simulink model "lo_values_test_v11"  (R2012b)
settings: Solver=ode45  StartTime=0.0  StopTime=100000  RelTol=1e-3
values from neighbouring files (symbols this model uses):
  Fs = 640e6    (= 640000000)    [filter_coefficients.m]    (also in filter_design.m; filter_design_getting_order.m)
undefined symbols (not defined in the file or in its folder): get, sided, Two
undefined symbols (not defined in the file): A_cos, A_sin, B_cos, B_sin, C_cos, C_sin, casper_coef, coef, D_cos, D_sin
libraries: xbsIndex_r4 x1768, dspsnks4 x10, casper_library_misc x9, xps_library x2, simulink x1
(part 2 of 17)

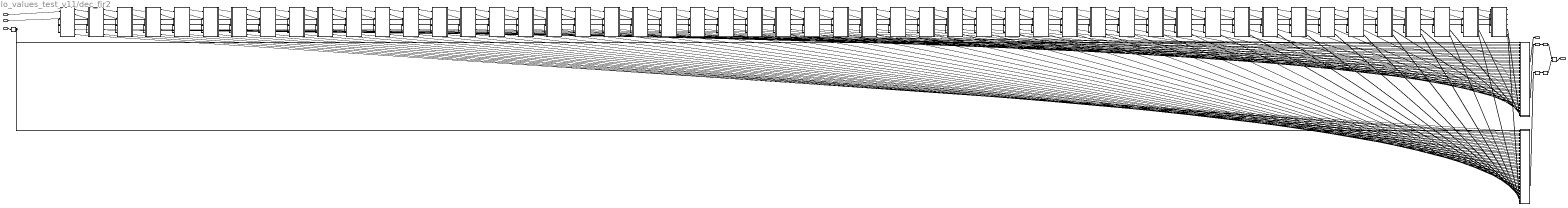
== system lo_values_test_v11/dec_fir2 ==
  sync_in : Inport
  real1 : Inport  Port=2
  imag1 : Inport  Port=3
  convert1 : xbsIndex_r4/Convert  gui_display_data_type=Fixed-point  arith_type="Signed  (2's comp)"  n_bits=16  bin_pt=15  float_type=Single  exp_bits=8  fraction_bits=24  quantization="Round  (unbiased: +/- Inf)"  overflow=Wrap  en=off  latency=2  dbl_ovrd=off  pipeline=off  block_type=convert
  convert2 : xbsIndex_r4/Convert  gui_display_data_type=Fixed-point  arith_type="Signed  (2's comp)"  n_bits=16  bin_pt=15  float_type=Single  exp_bits=8  fraction_bits=24  quantization="Round  (unbiased: +/- Inf)"  overflow=Wrap  en=off  latency=2  dbl_ovrd=off  pipeline=off  block_type=convert
  delay : xbsIndex_r4/Delay  rst=off  infoeditControl=Selection of Reset will increase slice count due to use of real FFs and instead of SRLs  en=off  latency=5  dbl_ovrd=off  reg_retiming=off  block_type=delay
  fir_dbl_col1 : Subsystem  AncestorBlock=casper_library_downconverter/fir_dbl_col  mask(fir_dbl_col){n_inputs=1, coeff=[0.00034504], add_latency=1, mult_latency=2, coeff_bit_width=25, coeff_bin_pt=24, first_stage_hdl=on, adder_imp=DSP48}
      mask prompts: n_inputs "Inputs"; coeff "Coefficients"; add_latency "Add latency"; mult_latency "Mult Latency"; coeff_bit_width "Coefficient bit width"; coeff_bin_pt "Coefficient binary point"; first_stage_hdl "Implement first stage of adder trees on output as behavioural HDL"; adder_imp "Adder implementation"
      mask init: same as lo_values_test_v11/dec_fir/fir_dbl_col1
      mask Help: eval('xlWeb(''http://casper.berkeley.edu/wiki/Fir_dbl_col'')')
      mask TypeOptions adder_imp: Behavioral | Fabric | DSP48
  fir_dbl_col10 : Subsystem  AncestorBlock=casper_library_downconverter/fir_dbl_col  mask(fir_dbl_col){n_inputs=1, coeff=[0.0011044], add_latency=1, mult_latency=2, coeff_bit_width=25, coeff_bin_pt=24, first_stage_hdl=on, adder_imp=DSP48}
      mask prompts: n_inputs "Inputs"; coeff "Coefficients"; add_latency "Add latency"; mult_latency "Mult Latency"; coeff_bit_width "Coefficient bit width"; coeff_bin_pt "Coefficient binary point"; first_stage_hdl "Implement first stage of adder trees on output as behavioural HDL"; adder_imp "Adder implementation"
      mask init: same as lo_values_test_v11/dec_fir/fir_dbl_col1
      mask Help: eval('xlWeb(''http://casper.berkeley.edu/wiki/Fir_dbl_col'')')
      mask TypeOptions adder_imp: Behavioral | Fabric | DSP48
  fir_dbl_col11 : Subsystem  AncestorBlock=casper_library_downconverter/fir_dbl_col  mask(fir_dbl_col){n_inputs=1, coeff=[0.0012861], add_latency=1, mult_latency=2, coeff_bit_width=25, coeff_bin_pt=24, first_stage_hdl=on, adder_imp=DSP48}
      mask prompts: n_inputs "Inputs"; coeff "Coefficients"; add_latency "Add latency"; mult_latency "Mult Latency"; coeff_bit_width "Coefficient bit width"; coeff_bin_pt "Coefficient binary point"; first_stage_hdl "Implement first stage of adder trees on output as behavioural HDL"; adder_imp "Adder implementation"
      mask init: same as lo_values_test_v11/dec_fir/fir_dbl_col1
      mask Help: eval('xlWeb(''http://casper.berkeley.edu/wiki/Fir_dbl_col'')')
      mask TypeOptions adder_imp: Behavioral | Fabric | DSP48
  fir_dbl_col12 : Subsystem  AncestorBlock=casper_library_downconverter/fir_dbl_col  mask(fir_dbl_col){n_inputs=1, coeff=[0.0014864], add_latency=1, mult_latency=2, coeff_bit_width=25, coeff_bin_pt=24, first_stage_hdl=on, adder_imp=DSP48}
      mask prompts: n_inputs "Inputs"; coeff "Coefficients"; add_latency "Add latency"; mult_latency "Mult Latency"; coeff_bit_width "Coefficient bit width"; coeff_bin_pt "Coefficient binary point"; first_stage_hdl "Implement first stage of adder trees on output as behavioural HDL"; adder_imp "Adder implementation"
      mask init: same as lo_values_test_v11/dec_fir/fir_dbl_col1
      mask Help: eval('xlWeb(''http://casper.berkeley.edu/wiki/Fir_dbl_col'')')
      mask TypeOptions adder_imp: Behavioral | Fabric | DSP48
  fir_dbl_col13 : Subsystem  AncestorBlock=casper_library_downconverter/fir_dbl_col  mask(fir_dbl_col){n_inputs=1, coeff=[0.0017056], add_latency=1, mult_latency=2, coeff_bit_width=25, coeff_bin_pt=24, first_stage_hdl=on, adder_imp=DSP48}
      mask prompts: n_inputs "Inputs"; coeff "Coefficients"; add_latency "Add latency"; mult_latency "Mult Latency"; coeff_bit_width "Coefficient bit width"; coeff_bin_pt "Coefficient binary point"; first_stage_hdl "Implement first stage of adder trees on output as behavioural HDL"; adder_imp "Adder implementation"
      mask init: same as lo_values_test_v11/dec_fir/fir_dbl_col1
      mask Help: eval('xlWeb(''http://casper.berkeley.edu/wiki/Fir_dbl_col'')')
      mask TypeOptions adder_imp: Behavioral | Fabric | DSP48
  fir_dbl_col14 : Subsystem  AncestorBlock=casper_library_downconverter/fir_dbl_col  mask(fir_dbl_col){n_inputs=1, coeff=[0.0019439], add_latency=1, mult_latency=2, coeff_bit_width=25, coeff_bin_pt=24, first_stage_hdl=on, adder_imp=DSP48}
      mask prompts: n_inputs "Inputs"; coeff "Coefficients"; add_latency "Add latency"; mult_latency "Mult Latency"; coeff_bit_width "Coefficient bit width"; coeff_bin_pt "Coefficient binary point"; first_stage_hdl "Implement first stage of adder trees on output as behavioural HDL"; adder_imp "Adder implementation"
      mask init: same as lo_values_test_v11/dec_fir/fir_dbl_col1
      mask Help: eval('xlWeb(''http://casper.berkeley.edu/wiki/Fir_dbl_col'')')
      mask TypeOptions adder_imp: Behavioral | Fabric | DSP48
  fir_dbl_col15 : Subsystem  AncestorBlock=casper_library_downconverter/fir_dbl_col  mask(fir_dbl_col){n_inputs=1, coeff=[0.0022021], add_latency=1, mult_latency=2, coeff_bit_width=25, coeff_bin_pt=24, first_stage_hdl=on, adder_imp=DSP48}
      mask prompts: n_inputs "Inputs"; coeff "Coefficients"; add_latency "Add latency"; mult_latency "Mult Latency"; coeff_bit_width "Coefficient bit width"; coeff_bin_pt "Coefficient binary point"; first_stage_hdl "Implement first stage of adder trees on output as behavioural HDL"; adder_imp "Adder implementation"
      mask init: same as lo_values_test_v11/dec_fir/fir_dbl_col1
      mask Help: eval('xlWeb(''http://casper.berkeley.edu/wiki/Fir_dbl_col'')')
      mask TypeOptions adder_imp: Behavioral | Fabric | DSP48
  fir_dbl_col16 : Subsystem  AncestorBlock=casper_library_downconverter/fir_dbl_col  mask(fir_dbl_col){n_inputs=1, coeff=[0.0024799], add_latency=1, mult_latency=2, coeff_bit_width=25, coeff_bin_pt=24, first_stage_hdl=on, adder_imp=DSP48}
      mask prompts: n_inputs "Inputs"; coeff "Coefficients"; add_latency "Add latency"; mult_latency "Mult Latency"; coeff_bit_width "Coefficient bit width"; coeff_bin_pt "Coefficient binary point"; first_stage_hdl "Implement first stage of adder trees on output as behavioural HDL"; adder_imp "Adder implementation"
      mask init: same as lo_values_test_v11/dec_fir/fir_dbl_col1
      mask Help: eval('xlWeb(''http://casper.berkeley.edu/wiki/Fir_dbl_col'')')
      mask TypeOptions adder_imp: Behavioral | Fabric | DSP48
  fir_dbl_col17 : Subsystem  AncestorBlock=casper_library_downconverter/fir_dbl_col  mask(fir_dbl_col){n_inputs=1, coeff=[0.0027778], add_latency=1, mult_latency=2, coeff_bit_width=25, coeff_bin_pt=24, first_stage_hdl=on, adder_imp=DSP48}
      mask prompts: n_inputs "Inputs"; coeff "Coefficients"; add_latency "Add latency"; mult_latency "Mult Latency"; coeff_bit_width "Coefficient bit width"; coeff_bin_pt "Coefficient binary point"; first_stage_hdl "Implement first stage of adder trees on output as behavioural HDL"; adder_imp "Adder implementation"
      mask init: same as lo_values_test_v11/dec_fir/fir_dbl_col1
      mask Help: eval('xlWeb(''http://casper.berkeley.edu/wiki/Fir_dbl_col'')')
      mask TypeOptions adder_imp: Behavioral | Fabric | DSP48
  fir_dbl_col18 : Subsystem  AncestorBlock=casper_library_downconverter/fir_dbl_col  mask(fir_dbl_col){n_inputs=1, coeff=[0.0030952], add_latency=1, mult_latency=2, coeff_bit_width=25, coeff_bin_pt=24, first_stage_hdl=on, adder_imp=DSP48}
      mask prompts: n_inputs "Inputs"; coeff "Coefficients"; add_latency "Add latency"; mult_latency "Mult Latency"; coeff_bit_width "Coefficient bit width"; coeff_bin_pt "Coefficient binary point"; first_stage_hdl "Implement first stage of adder trees on output as behavioural HDL"; adder_imp "Adder implementation"
      mask init: same as lo_values_test_v11/dec_fir/fir_dbl_col1
      mask Help: eval('xlWeb(''http://casper.berkeley.edu/wiki/Fir_dbl_col'')')
      mask TypeOptions adder_imp: Behavioral | Fabric | DSP48
  fir_dbl_col19 : Subsystem  AncestorBlock=casper_library_downconverter/fir_dbl_col  mask(fir_dbl_col){n_inputs=1, coeff=[0.0034322], add_latency=1, mult_latency=2, coeff_bit_width=25, coeff_bin_pt=24, first_stage_hdl=on, adder_imp=DSP48}
      mask prompts: n_inputs "Inputs"; coeff "Coefficients"; add_latency "Add latency"; mult_latency "Mult Latency"; coeff_bit_width "Coefficient bit width"; coeff_bin_pt "Coefficient binary point"; first_stage_hdl "Implement first stage of adder trees on output as behavioural HDL"; adder_imp "Adder implementation"
      mask init: same as lo_values_test_v11/dec_fir/fir_dbl_col1
      mask Help: eval('xlWeb(''http://casper.berkeley.edu/wiki/Fir_dbl_col'')')
      mask TypeOptions adder_imp: Behavioral | Fabric | DSP48
  fir_dbl_col2 : Subsystem  AncestorBlock=casper_library_downconverter/fir_dbl_col  mask(fir_dbl_col){n_inputs=1, coeff=[0.00021473], add_latency=1, mult_latency=2, coeff_bit_width=25, coeff_bin_pt=24, first_stage_hdl=on, adder_imp=DSP48}
      mask prompts: n_inputs "Inputs"; coeff "Coefficients"; add_latency "Add latency"; mult_latency "Mult Latency"; coeff_bit_width "Coefficient bit width"; coeff_bin_pt "Coefficient binary point"; first_stage_hdl "Implement first stage of adder trees on output as behavioural HDL"; adder_imp "Adder implementation"
      mask init: same as lo_values_test_v11/dec_fir/fir_dbl_col1
      mask Help: eval('xlWeb(''http://casper.berkeley.edu/wiki/Fir_dbl_col'')')
      mask TypeOptions adder_imp: Behavioral | Fabric | DSP48
  fir_dbl_col20 : Subsystem  AncestorBlock=casper_library_downconverter/fir_dbl_col  mask(fir_dbl_col){n_inputs=1, coeff=[0.003788], add_latency=1, mult_latency=2, coeff_bit_width=25, coeff_bin_pt=24, first_stage_hdl=on, adder_imp=DSP48}
      mask prompts: n_inputs "Inputs"; coeff "Coefficients"; add_latency "Add latency"; mult_latency "Mult Latency"; coeff_bit_width "Coefficient bit width"; coeff_bin_pt "Coefficient binary point"; first_stage_hdl "Implement first stage of adder trees on output as behavioural HDL"; adder_imp "Adder implementation"
      mask init: same as lo_values_test_v11/dec_fir/fir_dbl_col1
      mask Help: eval('xlWeb(''http://casper.berkeley.edu/wiki/Fir_dbl_col'')')
      mask TypeOptions adder_imp: Behavioral | Fabric | DSP48
  fir_dbl_col21 : Subsystem  AncestorBlock=casper_library_downconverter/fir_dbl_col  mask(fir_dbl_col){n_inputs=1, coeff=[0.0041621], add_latency=1, mult_latency=2, coeff_bit_width=25, coeff_bin_pt=24, first_stage_hdl=on, adder_imp=DSP48}
      mask prompts: n_inputs "Inputs"; coeff "Coefficients"; add_latency "Add latency"; mult_latency "Mult Latency"; coeff_bit_width "Coefficient bit width"; coeff_bin_pt "Coefficient binary point"; first_stage_hdl "Implement first stage of adder trees on output as behavioural HDL"; adder_imp "Adder implementation"
      mask init: same as lo_values_test_v11/dec_fir/fir_dbl_col1
      mask Help: eval('xlWeb(''http://casper.berkeley.edu/wiki/Fir_dbl_col'')')
      mask TypeOptions adder_imp: Behavioral | Fabric | DSP48
  fir_dbl_col22 : Subsystem  AncestorBlock=casper_library_downconverter/fir_dbl_col  mask(fir_dbl_col){n_inputs=1, coeff=[0.0045537], add_latency=1, mult_latency=2, coeff_bit_width=25, coeff_bin_pt=24, first_stage_hdl=on, adder_imp=DSP48}
      mask prompts: n_inputs "Inputs"; coeff "Coefficients"; add_latency "Add latency"; mult_latency "Mult Latency"; coeff_bit_width "Coefficient bit width"; coeff_bin_pt "Coefficient binary point"; first_stage_hdl "Implement first stage of adder trees on output as behavioural HDL"; adder_imp "Adder implementation"
      mask init: same as lo_values_test_v11/dec_fir/fir_dbl_col1
      mask Help: eval('xlWeb(''http://casper.berkeley.edu/wiki/Fir_dbl_col'')')
      mask TypeOptions adder_imp: Behavioral | Fabric | DSP48
  fir_dbl_col23 : Subsystem  AncestorBlock=casper_library_downconverter/fir_dbl_col  mask(fir_dbl_col){n_inputs=1, coeff=[0.0049616], add_latency=1, mult_latency=2, coeff_bit_width=25, coeff_bin_pt=24, first_stage_hdl=on, adder_imp=DSP48}
      mask prompts: n_inputs "Inputs"; coeff "Coefficients"; add_latency "Add latency"; mult_latency "Mult Latency"; coeff_bit_width "Coefficient bit width"; coeff_bin_pt "Coefficient binary point"; first_stage_hdl "Implement first stage of adder trees on output as behavioural HDL"; adder_imp "Adder implementation"
      mask init: same as lo_values_test_v11/dec_fir/fir_dbl_col1
      mask Help: eval('xlWeb(''http://casper.berkeley.edu/wiki/Fir_dbl_col'')')
      mask TypeOptions adder_imp: Behavioral | Fabric | DSP48
  fir_dbl_col24 : Subsystem  AncestorBlock=casper_library_downconverter/fir_dbl_col  mask(fir_dbl_col){n_inputs=1, coeff=[0.0053848], add_latency=1, mult_latency=2, coeff_bit_width=25, coeff_bin_pt=24, first_stage_hdl=on, adder_imp=DSP48}
      mask prompts: n_inputs "Inputs"; coeff "Coefficients"; add_latency "Add latency"; mult_latency "Mult Latency"; coeff_bit_width "Coefficient bit width"; coeff_bin_pt "Coefficient binary point"; first_stage_hdl "Implement first stage of adder trees on output as behavioural HDL"; adder_imp "Adder implementation"
      mask init: same as lo_values_test_v11/dec_fir/fir_dbl_col1
      mask Help: eval('xlWeb(''http://casper.berkeley.edu/wiki/Fir_dbl_col'')')
      mask TypeOptions adder_imp: Behavioral | Fabric | DSP48
  fir_dbl_col25 : Subsystem  AncestorBlock=casper_library_downconverter/fir_dbl_col  mask(fir_dbl_col){n_inputs=1, coeff=[0.0058219], add_latency=1, mult_latency=2, coeff_bit_width=25, coeff_bin_pt=24, first_stage_hdl=on, adder_imp=DSP48}
      mask prompts: n_inputs "Inputs"; coeff "Coefficients"; add_latency "Add latency"; mult_latency "Mult Latency"; coeff_bit_width "Coefficient bit width"; coeff_bin_pt "Coefficient binary point"; first_stage_hdl "Implement first stage of adder trees on output as behavioural HDL"; adder_imp "Adder implementation"
      mask init: same as lo_values_test_v11/dec_fir/fir_dbl_col1
      mask Help: eval('xlWeb(''http://casper.berkeley.edu/wiki/Fir_dbl_col'')')
      mask TypeOptions adder_imp: Behavioral | Fabric | DSP48
  fir_dbl_col26 : Subsystem  AncestorBlock=casper_library_downconverter/fir_dbl_col  mask(fir_dbl_col){n_inputs=1, coeff=[0.0062713], add_latency=1, mult_latency=2, coeff_bit_width=25, coeff_bin_pt=24, first_stage_hdl=on, adder_imp=DSP48}
      mask prompts: n_inputs "Inputs"; coeff "Coefficients"; add_latency "Add latency"; mult_latency "Mult Latency"; coeff_bit_width "Coefficient bit width"; coeff_bin_pt "Coefficient binary point"; first_stage_hdl "Implement first stage of adder trees on output as behavioural HDL"; adder_imp "Adder implementation"
      mask init: same as lo_values_test_v11/dec_fir/fir_dbl_col1
      mask Help: eval('xlWeb(''http://casper.berkeley.edu/wiki/Fir_dbl_col'')')
      mask TypeOptions adder_imp: Behavioral | Fabric | DSP48
  fir_dbl_col27 : Subsystem  AncestorBlock=casper_library_downconverter/fir_dbl_col  mask(fir_dbl_col){n_inputs=1, coeff=[0.0067313], add_latency=1, mult_latency=2, coeff_bit_width=25, coeff_bin_pt=24, first_stage_hdl=on, adder_imp=DSP48}
      mask prompts: n_inputs "Inputs"; coeff "Coefficients"; add_latency "Add latency"; mult_latency "Mult Latency"; coeff_bit_width "Coefficient bit width"; coeff_bin_pt "Coefficient binary point"; first_stage_hdl "Implement first stage of adder trees on output as behavioural HDL"; adder_imp "Adder implementation"
      mask init: same as lo_values_test_v11/dec_fir/fir_dbl_col1
      mask Help: eval('xlWeb(''http://casper.berkeley.edu/wiki/Fir_dbl_col'')')
      mask TypeOptions adder_imp: Behavioral | Fabric | DSP48
  fir_dbl_col28 : Subsystem  AncestorBlock=casper_library_downconverter/fir_dbl_col  mask(fir_dbl_col){n_inputs=1, coeff=[0.0072001], add_latency=1, mult_latency=2, coeff_bit_width=25, coeff_bin_pt=24, first_stage_hdl=on, adder_imp=DSP48}
      mask prompts: n_inputs "Inputs"; coeff "Coefficients"; add_latency "Add latency"; mult_latency "Mult Latency"; coeff_bit_width "Coefficient bit width"; coeff_bin_pt "Coefficient binary point"; first_stage_hdl "Implement first stage of adder trees on output as behavioural HDL"; adder_imp "Adder implementation"
      mask init: same as lo_values_test_v11/dec_fir/fir_dbl_col1
      mask Help: eval('xlWeb(''http://casper.berkeley.edu/wiki/Fir_dbl_col'')')
      mask TypeOptions adder_imp: Behavioral | Fabric | DSP48
  fir_dbl_col29 : Subsystem  AncestorBlock=casper_library_downconverter/fir_dbl_col  mask(fir_dbl_col){n_inputs=1, coeff=[0.0076755], add_latency=1, mult_latency=2, coeff_bit_width=25, coeff_bin_pt=24, first_stage_hdl=on, adder_imp=DSP48}
      mask prompts: n_inputs "Inputs"; coeff "Coefficients"; add_latency "Add latency"; mult_latency "Mult Latency"; coeff_bit_width "Coefficient bit width"; coeff_bin_pt "Coefficient binary point"; first_stage_hdl "Implement first stage of adder trees on output as behavioural HDL"; adder_imp "Adder implementation"
      mask init: same as lo_values_test_v11/dec_fir/fir_dbl_col1
      mask Help: eval('xlWeb(''http://casper.berkeley.edu/wiki/Fir_dbl_col'')')
      mask TypeOptions adder_imp: Behavioral | Fabric | DSP48
  fir_dbl_col3 : Subsystem  AncestorBlock=casper_library_downconverter/fir_dbl_col  mask(fir_dbl_col){n_inputs=1, coeff=[0.00027945], add_latency=1, mult_latency=2, coeff_bit_width=25, coeff_bin_pt=24, first_stage_hdl=on, adder_imp=DSP48}
      mask prompts: n_inputs "Inputs"; coeff "Coefficients"; add_latency "Add latency"; mult_latency "Mult Latency"; coeff_bit_width "Coefficient bit width"; coeff_bin_pt "Coefficient binary point"; first_stage_hdl "Implement first stage of adder trees on output as behavioural HDL"; adder_imp "Adder implementation"
      mask init: same as lo_values_test_v11/dec_fir/fir_dbl_col1
      mask Help: eval('xlWeb(''http://casper.berkeley.edu/wiki/Fir_dbl_col'')')
      mask TypeOptions adder_imp: Behavioral | Fabric | DSP48
  fir_dbl_col30 : Subsystem  AncestorBlock=casper_library_downconverter/fir_dbl_col  mask(fir_dbl_col){n_inputs=1, coeff=[0.0081554], add_latency=1, mult_latency=2, coeff_bit_width=25, coeff_bin_pt=24, first_stage_hdl=on, adder_imp=DSP48}
      mask prompts: n_inputs "Inputs"; coeff "Coefficients"; add_latency "Add latency"; mult_latency "Mult Latency"; coeff_bit_width "Coefficient bit width"; coeff_bin_pt "Coefficient binary point"; first_stage_hdl "Implement first stage of adder trees on output as behavioural HDL"; adder_imp "Adder implementation"
      mask init: same as lo_values_test_v11/dec_fir/fir_dbl_col1
      mask Help: eval('xlWeb(''http://casper.berkeley.edu/wiki/Fir_dbl_col'')')
      mask TypeOptions adder_imp: Behavioral | Fabric | DSP48
  fir_dbl_col31 : Subsystem  AncestorBlock=casper_library_downconverter/fir_dbl_col  mask(fir_dbl_col){n_inputs=1, coeff=[0.0086376], add_latency=1, mult_latency=2, coeff_bit_width=25, coeff_bin_pt=24, first_stage_hdl=on, adder_imp=DSP48}
      mask prompts: n_inputs "Inputs"; coeff "Coefficients"; add_latency "Add latency"; mult_latency "Mult Latency"; coeff_bit_width "Coefficient bit width"; coeff_bin_pt "Coefficient binary point"; first_stage_hdl "Implement first stage of adder trees on output as behavioural HDL"; adder_imp "Adder implementation"
      mask init: same as lo_values_test_v11/dec_fir/fir_dbl_col1
      mask Help: eval('xlWeb(''http://casper.berkeley.edu/wiki/Fir_dbl_col'')')
      mask TypeOptions adder_imp: Behavioral | Fabric | DSP48
  fir_dbl_col32 : Subsystem  AncestorBlock=casper_library_downconverter/fir_dbl_col  mask(fir_dbl_col){n_inputs=1, coeff=[0.0091195], add_latency=1, mult_latency=2, coeff_bit_width=25, coeff_bin_pt=24, first_stage_hdl=on, adder_imp=DSP48}
      mask prompts: n_inputs "Inputs"; coeff "Coefficients"; add_latency "Add latency"; mult_latency "Mult Latency"; coeff_bit_width "Coefficient bit width"; coeff_bin_pt "Coefficient binary point"; first_stage_hdl "Implement first stage of adder trees on output as behavioural HDL"; adder_imp "Adder implementation"
      mask init: same as lo_values_test_v11/dec_fir/fir_dbl_col1
      mask Help: eval('xlWeb(''http://casper.berkeley.edu/wiki/Fir_dbl_col'')')
      mask TypeOptions adder_imp: Behavioral | Fabric | DSP48
  fir_dbl_col33 : Subsystem  AncestorBlock=casper_library_downconverter/fir_dbl_col  mask(fir_dbl_col){n_inputs=1, coeff=[0.009599], add_latency=1, mult_latency=2, coeff_bit_width=25, coeff_bin_pt=24, first_stage_hdl=on, adder_imp=DSP48}
      mask prompts: n_inputs "Inputs"; coeff "Coefficients"; add_latency "Add latency"; mult_latency "Mult Latency"; coeff_bit_width "Coefficient bit width"; coeff_bin_pt "Coefficient binary point"; first_stage_hdl "Implement first stage of adder trees on output as behavioural HDL"; adder_imp "Adder implementation"
      mask init: same as lo_values_test_v11/dec_fir/fir_dbl_col1
      mask Help: eval('xlWeb(''http://casper.berkeley.edu/wiki/Fir_dbl_col'')')
      mask TypeOptions adder_imp: Behavioral | Fabric | DSP48
  fir_dbl_col34 : Subsystem  AncestorBlock=casper_library_downconverter/fir_dbl_col  mask(fir_dbl_col){n_inputs=1, coeff=[0.010073], add_latency=1, mult_latency=2, coeff_bit_width=25, coeff_bin_pt=24, first_stage_hdl=on, adder_imp=DSP48}
      mask prompts: n_inputs "Inputs"; coeff "Coefficients"; add_latency "Add latency"; mult_latency "Mult Latency"; coeff_bit_width "Coefficient bit width"; coeff_bin_pt "Coefficient binary point"; first_stage_hdl "Implement first stage of adder trees on output as behavioural HDL"; adder_imp "Adder implementation"
      mask init: same as lo_values_test_v11/dec_fir/fir_dbl_col1
      mask Help: eval('xlWeb(''http://casper.berkeley.edu/wiki/Fir_dbl_col'')')
      mask TypeOptions adder_imp: Behavioral | Fabric | DSP48
  fir_dbl_col35 : Subsystem  AncestorBlock=casper_library_downconverter/fir_dbl_col  mask(fir_dbl_col){n_inputs=1, coeff=[0.01054], add_latency=1, mult_latency=2, coeff_bit_width=25, coeff_bin_pt=24, first_stage_hdl=on, adder_imp=DSP48}
      mask prompts: n_inputs "Inputs"; coeff "Coefficients"; add_latency "Add latency"; mult_latency "Mult Latency"; coeff_bit_width "Coefficient bit width"; coeff_bin_pt "Coefficient binary point"; first_stage_hdl "Implement first stage of adder trees on output as behavioural HDL"; adder_imp "Adder implementation"
      mask init: same as lo_values_test_v11/dec_fir/fir_dbl_col1
      mask Help: eval('xlWeb(''http://casper.berkeley.edu/wiki/Fir_dbl_col'')')
      mask TypeOptions adder_imp: Behavioral | Fabric | DSP48
  fir_dbl_col36 : Subsystem  AncestorBlock=casper_library_downconverter/fir_dbl_col  mask(fir_dbl_col){n_inputs=1, coeff=[0.010996], add_latency=1, mult_latency=2, coeff_bit_width=25, coeff_bin_pt=24, first_stage_hdl=on, adder_imp=DSP48}
      mask prompts: n_inputs "Inputs"; coeff "Coefficients"; add_latency "Add latency"; mult_latency "Mult Latency"; coeff_bit_width "Coefficient bit width"; coeff_bin_pt "Coefficient binary point"; first_stage_hdl "Implement first stage of adder trees on output as behavioural HDL"; adder_imp "Adder implementation"
      mask init: same as lo_values_test_v11/dec_fir/fir_dbl_col1
      mask Help: eval('xlWeb(''http://casper.berkeley.edu/wiki/Fir_dbl_col'')')
      mask TypeOptions adder_imp: Behavioral | Fabric | DSP48
  fir_dbl_col37 : Subsystem  AncestorBlock=casper_library_downconverter/fir_dbl_col  mask(fir_dbl_col){n_inputs=1, coeff=[0.011439], add_latency=1, mult_latency=2, coeff_bit_width=25, coeff_bin_pt=24, first_stage_hdl=on, adder_imp=DSP48}
      mask prompts: n_inputs "Inputs"; coeff "Coefficients"; add_latency "Add latency"; mult_latency "Mult Latency"; coeff_bit_width "Coefficient bit width"; coeff_bin_pt "Coefficient binary point"; first_stage_hdl "Implement first stage of adder trees on output as behavioural HDL"; adder_imp "Adder implementation"
      mask init: same as lo_values_test_v11/dec_fir/fir_dbl_col1
      mask Help: eval('xlWeb(''http://casper.berkeley.edu/wiki/Fir_dbl_col'')')
      mask TypeOptions adder_imp: Behavioral | Fabric | DSP48
  fir_dbl_col38 : Subsystem  AncestorBlock=casper_library_downconverter/fir_dbl_col  mask(fir_dbl_col){n_inputs=1, coeff=[0.011867], add_latency=1, mult_latency=2, coeff_bit_width=25, coeff_bin_pt=24, first_stage_hdl=on, adder_imp=DSP48}
      mask prompts: n_inputs "Inputs"; coeff "Coefficients"; add_latency "Add latency"; mult_latency "Mult Latency"; coeff_bit_width "Coefficient bit width"; coeff_bin_pt "Coefficient binary point"; first_stage_hdl "Implement first stage of adder trees on output as behavioural HDL"; adder_imp "Adder implementation"
      mask init: same as lo_values_test_v11/dec_fir/fir_dbl_col1
      mask Help: eval('xlWeb(''http://casper.berkeley.edu/wiki/Fir_dbl_col'')')
      mask TypeOptions adder_imp: Behavioral | Fabric | DSP48
  fir_dbl_col39 : Subsystem  AncestorBlock=casper_library_downconverter/fir_dbl_col  mask(fir_dbl_col){n_inputs=1, coeff=[0.012277], add_latency=1, mult_latency=2, coeff_bit_width=25, coeff_bin_pt=24, first_stage_hdl=on, adder_imp=DSP48}
      mask prompts: n_inputs "Inputs"; coeff "Coefficients"; add_latency "Add latency"; mult_latency "Mult Latency"; coeff_bit_width "Coefficient bit width"; coeff_bin_pt "Coefficient binary point"; first_stage_hdl "Implement first stage of adder trees on output as behavioural HDL"; adder_imp "Adder implementation"
      mask init: same as lo_values_test_v11/dec_fir/fir_dbl_col1
      mask Help: eval('xlWeb(''http://casper.berkeley.edu/wiki/Fir_dbl_col'')')
      mask TypeOptions adder_imp: Behavioral | Fabric | DSP48
  fir_dbl_col4 : Subsystem  AncestorBlock=casper_library_downconverter/fir_dbl_col  mask(fir_dbl_col){n_inputs=1, coeff=[0.00035551], add_latency=1, mult_latency=2, coeff_bit_width=25, coeff_bin_pt=24, first_stage_hdl=on, adder_imp=DSP48}
      mask prompts: n_inputs "Inputs"; coeff "Coefficients"; add_latency "Add latency"; mult_latency "Mult Latency"; coeff_bit_width "Coefficient bit width"; coeff_bin_pt "Coefficient binary point"; first_stage_hdl "Implement first stage of adder trees on output as behavioural HDL"; adder_imp "Adder implementation"
      mask init: same as lo_values_test_v11/dec_fir/fir_dbl_col1
      mask Help: eval('xlWeb(''http://casper.berkeley.edu/wiki/Fir_dbl_col'')')
      mask TypeOptions adder_imp: Behavioral | Fabric | DSP48
  fir_dbl_col40 : Subsystem  AncestorBlock=casper_library_downconverter/fir_dbl_col  mask(fir_dbl_col){n_inputs=1, coeff=[0.012666], add_latency=1, mult_latency=2, coeff_bit_width=25, coeff_bin_pt=24, first_stage_hdl=on, adder_imp=DSP48}
      mask prompts: n_inputs "Inputs"; coeff "Coefficients"; add_latency "Add latency"; mult_latency "Mult Latency"; coeff_bit_width "Coefficient bit width"; coeff_bin_pt "Coefficient binary point"; first_stage_hdl "Implement first stage of adder trees on output as behavioural HDL"; adder_imp "Adder implementation"
      mask init: same as lo_values_test_v11/dec_fir/fir_dbl_col1
      mask Help: eval('xlWeb(''http://casper.berkeley.edu/wiki/Fir_dbl_col'')')
      mask TypeOptions adder_imp: Behavioral | Fabric | DSP48
  fir_dbl_col41 : Subsystem  AncestorBlock=casper_library_downconverter/fir_dbl_col  mask(fir_dbl_col){n_inputs=1, coeff=[0.013032], add_latency=1, mult_latency=2, coeff_bit_width=25, coeff_bin_pt=24, first_stage_hdl=on, adder_imp=DSP48}
      mask prompts: n_inputs "Inputs"; coeff "Coefficients"; add_latency "Add latency"; mult_latency "Mult Latency"; coeff_bit_width "Coefficient bit width"; coeff_bin_pt "Coefficient binary point"; first_stage_hdl "Implement first stage of adder trees on output as behavioural HDL"; adder_imp "Adder implementation"
      mask init: same as lo_values_test_v11/dec_fir/fir_dbl_col1
      mask Help: eval('xlWeb(''http://casper.berkeley.edu/wiki/Fir_dbl_col'')')
      mask TypeOptions adder_imp: Behavioral | Fabric | DSP48
  fir_dbl_col42 : Subsystem  AncestorBlock=casper_library_downconverter/fir_dbl_col  mask(fir_dbl_col){n_inputs=1, coeff=[0.013373], add_latency=1, mult_latency=2, coeff_bit_width=25, coeff_bin_pt=24, first_stage_hdl=on, adder_imp=DSP48}
      mask prompts: n_inputs "Inputs"; coeff "Coefficients"; add_latency "Add latency"; mult_latency "Mult Latency"; coeff_bit_width "Coefficient bit width"; coeff_bin_pt "Coefficient binary point"; first_stage_hdl "Implement first stage of adder trees on output as behavioural HDL"; adder_imp "Adder implementation"
      mask init: same as lo_values_test_v11/dec_fir/fir_dbl_col1
      mask Help: eval('xlWeb(''http://casper.berkeley.edu/wiki/Fir_dbl_col'')')
      mask TypeOptions adder_imp: Behavioral | Fabric | DSP48
  fir_dbl_col43 : Subsystem  AncestorBlock=casper_library_downconverter/fir_dbl_col  mask(fir_dbl_col){n_inputs=1, coeff=[0.013686], add_latency=1, mult_latency=2, coeff_bit_width=25, coeff_bin_pt=24, first_stage_hdl=on, adder_imp=DSP48}
      mask prompts: n_inputs "Inputs"; coeff "Coefficients"; add_latency "Add latency"; mult_latency "Mult Latency"; coeff_bit_width "Coefficient bit width"; coeff_bin_pt "Coefficient binary point"; first_stage_hdl "Implement first stage of adder trees on output as behavioural HDL"; adder_imp "Adder implementation"
      mask init: same as lo_values_test_v11/dec_fir/fir_dbl_col1
      mask Help: eval('xlWeb(''http://casper.berkeley.edu/wiki/Fir_dbl_col'')')
      mask TypeOptions adder_imp: Behavioral | Fabric | DSP48
  fir_dbl_col44 : Subsystem  AncestorBlock=casper_library_downconverter/fir_dbl_col  mask(fir_dbl_col){n_inputs=1, coeff=[0.01397], add_latency=1, mult_latency=2, coeff_bit_width=25, coeff_bin_pt=24, first_stage_hdl=on, adder_imp=DSP48}
      mask prompts: n_inputs "Inputs"; coeff "Coefficients"; add_latency "Add latency"; mult_latency "Mult Latency"; coeff_bit_width "Coefficient bit width"; coeff_bin_pt "Coefficient binary point"; first_stage_hdl "Implement first stage of adder trees on output as behavioural HDL"; adder_imp "Adder implementation"
      mask init: same as lo_values_test_v11/dec_fir/fir_dbl_col1
      mask Help: eval('xlWeb(''http://casper.berkeley.edu/wiki/Fir_dbl_col'')')
      mask TypeOptions adder_imp: Behavioral | Fabric | DSP48
  fir_dbl_col45 : Subsystem  AncestorBlock=casper_library_downconverter/fir_dbl_col  mask(fir_dbl_col){n_inputs=1, coeff=[0.014223], add_latency=1, mult_latency=2, coeff_bit_width=25, coeff_bin_pt=24, first_stage_hdl=on, adder_imp=DSP48}
      mask prompts: n_inputs "Inputs"; coeff "Coefficients"; add_latency "Add latency"; mult_latency "Mult Latency"; coeff_bit_width "Coefficient bit width"; coeff_bin_pt "Coefficient binary point"; first_stage_hdl "Implement first stage of adder trees on output as behavioural HDL"; adder_imp "Adder implementation"
      mask init: same as lo_values_test_v11/dec_fir/fir_dbl_col1
      mask Help: eval('xlWeb(''http://casper.berkeley.edu/wiki/Fir_dbl_col'')')
      mask TypeOptions adder_imp: Behavioral | Fabric | DSP48
  fir_dbl_col46 : Subsystem  AncestorBlock=casper_library_downconverter/fir_dbl_col  mask(fir_dbl_col){n_inputs=1, coeff=[0.014442], add_latency=1, mult_latency=2, coeff_bit_width=25, coeff_bin_pt=24, first_stage_hdl=on, adder_imp=DSP48}
      mask prompts: n_inputs "Inputs"; coeff "Coefficients"; add_latency "Add latency"; mult_latency "Mult Latency"; coeff_bit_width "Coefficient bit width"; coeff_bin_pt "Coefficient binary point"; first_stage_hdl "Implement first stage of adder trees on output as behavioural HDL"; adder_imp "Adder implementation"
      mask init: same as lo_values_test_v11/dec_fir/fir_dbl_col1
      mask Help: eval('xlWeb(''http://casper.berkeley.edu/wiki/Fir_dbl_col'')')
      mask TypeOptions adder_imp: Behavioral | Fabric | DSP48
  fir_dbl_col47 : Subsystem  AncestorBlock=casper_library_downconverter/fir_dbl_col  mask(fir_dbl_col){n_inputs=1, coeff=[0.014628], add_latency=1, mult_latency=2, coeff_bit_width=25, coeff_bin_pt=24, first_stage_hdl=on, adder_imp=DSP48}
      mask prompts: n_inputs "Inputs"; coeff "Coefficients"; add_latency "Add latency"; mult_latency "Mult Latency"; coeff_bit_width "Coefficient bit width"; coeff_bin_pt "Coefficient binary point"; first_stage_hdl "Implement first stage of adder trees on output as behavioural HDL"; adder_imp "Adder implementation"
      mask init: same as lo_values_test_v11/dec_fir/fir_dbl_col1
      mask Help: eval('xlWeb(''http://casper.berkeley.edu/wiki/Fir_dbl_col'')')
      mask TypeOptions adder_imp: Behavioral | Fabric | DSP48
  fir_dbl_col48 : Subsystem  AncestorBlock=casper_library_downconverter/fir_dbl_col  mask(fir_dbl_col){n_inputs=1, coeff=[0.014778], add_latency=1, mult_latency=2, coeff_bit_width=25, coeff_bin_pt=24, first_stage_hdl=on, adder_imp=DSP48}
      mask prompts: n_inputs "Inputs"; coeff "Coefficients"; add_latency "Add latency"; mult_latency "Mult Latency"; coeff_bit_width "Coefficient bit width"; coeff_bin_pt "Coefficient binary point"; first_stage_hdl "Implement first stage of adder trees on output as behavioural HDL"; adder_imp "Adder implementation"
      mask init: same as lo_values_test_v11/dec_fir/fir_dbl_col1
      mask Help: eval('xlWeb(''http://casper.berkeley.edu/wiki/Fir_dbl_col'')')
      mask TypeOptions adder_imp: Behavioral | Fabric | DSP48
  fir_dbl_col49 : Subsystem  AncestorBlock=casper_library_downconverter/fir_dbl_col  mask(fir_dbl_col){n_inputs=1, coeff=[0.014891], add_latency=1, mult_latency=2, coeff_bit_width=25, coeff_bin_pt=24, first_stage_hdl=on, adder_imp=DSP48}
      mask prompts: n_inputs "Inputs"; coeff "Coefficients"; add_latency "Add latency"; mult_latency "Mult Latency"; coeff_bit_width "Coefficient bit width"; coeff_bin_pt "Coefficient binary point"; first_stage_hdl "Implement first stage of adder trees on output as behavioural HDL"; adder_imp "Adder implementation"
      mask init: same as lo_values_test_v11/dec_fir/fir_dbl_col1
      mask Help: eval('xlWeb(''http://casper.berkeley.edu/wiki/Fir_dbl_col'')')
      mask TypeOptions adder_imp: Behavioral | Fabric | DSP48
  fir_dbl_col5 : Subsystem  AncestorBlock=casper_library_downconverter/fir_dbl_col  mask(fir_dbl_col){n_inputs=1, coeff=[0.00044384], add_latency=1, mult_latency=2, coeff_bit_width=25, coeff_bin_pt=24, first_stage_hdl=on, adder_imp=DSP48}
      mask prompts: n_inputs "Inputs"; coeff "Coefficients"; add_latency "Add latency"; mult_latency "Mult Latency"; coeff_bit_width "Coefficient bit width"; coeff_bin_pt "Coefficient binary point"; first_stage_hdl "Implement first stage of adder trees on output as behavioural HDL"; adder_imp "Adder implementation"
      mask init: same as lo_values_test_v11/dec_fir/fir_dbl_col1
      mask Help: eval('xlWeb(''http://casper.berkeley.edu/wiki/Fir_dbl_col'')')
      mask TypeOptions adder_imp: Behavioral | Fabric | DSP48
  fir_dbl_col50 : Subsystem  AncestorBlock=casper_library_downconverter/fir_dbl_col  mask(fir_dbl_col){n_inputs=1, coeff=[0.014967], add_latency=1, mult_latency=2, coeff_bit_width=25, coeff_bin_pt=24, first_stage_hdl=on, adder_imp=DSP48}
      mask prompts: n_inputs "Inputs"; coeff "Coefficients"; add_latency "Add latency"; mult_latency "Mult Latency"; coeff_bit_width "Coefficient bit width"; coeff_bin_pt "Coefficient binary point"; first_stage_hdl "Implement first stage of adder trees on output as behavioural HDL"; adder_imp "Adder implementation"
      mask init: same as lo_values_test_v11/dec_fir/fir_dbl_col1
      mask Help: eval('xlWeb(''http://casper.berkeley.edu/wiki/Fir_dbl_col'')')
      mask TypeOptions adder_imp: Behavioral | Fabric | DSP48
  fir_dbl_col51 : Subsystem  AncestorBlock=casper_library_downconverter/fir_dbl_col  mask(fir_dbl_col){n_inputs=1, coeff=[0.015005], add_latency=1, mult_latency=2, coeff_bit_width=25, coeff_bin_pt=24, first_stage_hdl=on, adder_imp=DSP48}
      mask prompts: n_inputs "Inputs"; coeff "Coefficients"; add_latency "Add latency"; mult_latency "Mult Latency"; coeff_bit_width "Coefficient bit width"; coeff_bin_pt "Coefficient binary point"; first_stage_hdl "Implement first stage of adder trees on output as behavioural HDL"; adder_imp "Adder implementation"
      mask init: same as lo_values_test_v11/dec_fir/fir_dbl_col1
      mask Help: eval('xlWeb(''http://casper.berkeley.edu/wiki/Fir_dbl_col'')')
      mask TypeOptions adder_imp: Behavioral | Fabric | DSP48
  fir_dbl_col6 : Subsystem  AncestorBlock=casper_library_downconverter/fir_dbl_col  mask(fir_dbl_col){n_inputs=1, coeff=[0.00054573], add_latency=1, mult_latency=2, coeff_bit_width=25, coeff_bin_pt=24, first_stage_hdl=on, adder_imp=DSP48}
      mask prompts: n_inputs "Inputs"; coeff "Coefficients"; add_latency "Add latency"; mult_latency "Mult Latency"; coeff_bit_width "Coefficient bit width"; coeff_bin_pt "Coefficient binary point"; first_stage_hdl "Implement first stage of adder trees on output as behavioural HDL"; adder_imp "Adder implementation"
      mask init: same as lo_values_test_v11/dec_fir/fir_dbl_col1
      mask Help: eval('xlWeb(''http://casper.berkeley.edu/wiki/Fir_dbl_col'')')
      mask TypeOptions adder_imp: Behavioral | Fabric | DSP48
  fir_dbl_col7 : Subsystem  AncestorBlock=casper_library_downconverter/fir_dbl_col  mask(fir_dbl_col){n_inputs=1, coeff=[0.00066171], add_latency=1, mult_latency=2, coeff_bit_width=25, coeff_bin_pt=24, first_stage_hdl=on, adder_imp=DSP48}
      mask prompts: n_inputs "Inputs"; coeff "Coefficients"; add_latency "Add latency"; mult_latency "Mult Latency"; coeff_bit_width "Coefficient bit width"; coeff_bin_pt "Coefficient binary point"; first_stage_hdl "Implement first stage of adder trees on output as behavioural HDL"; adder_imp "Adder implementation"
      mask init: same as lo_values_test_v11/dec_fir/fir_dbl_col1
      mask Help: eval('xlWeb(''http://casper.berkeley.edu/wiki/Fir_dbl_col'')')
      mask TypeOptions adder_imp: Behavioral | Fabric | DSP48
  fir_dbl_col8 : Subsystem  AncestorBlock=casper_library_downconverter/fir_dbl_col  mask(fir_dbl_col){n_inputs=1, coeff=[0.00079278], add_latency=1, mult_latency=2, coeff_bit_width=25, coeff_bin_pt=24, first_stage_hdl=on, adder_imp=DSP48}
      mask prompts: n_inputs "Inputs"; coeff "Coefficients"; add_latency "Add latency"; mult_latency "Mult Latency"; coeff_bit_width "Coefficient bit width"; coeff_bin_pt "Coefficient binary point"; first_stage_hdl "Implement first stage of adder trees on output as behavioural HDL"; adder_imp "Adder implementation"
      mask init: same as lo_values_test_v11/dec_fir/fir_dbl_col1
      mask Help: eval('xlWeb(''http://casper.berkeley.edu/wiki/Fir_dbl_col'')')
      mask TypeOptions adder_imp: Behavioral | Fabric | DSP48
  fir_dbl_col9 : Subsystem  AncestorBlock=casper_library_downconverter/fir_dbl_col  mask(fir_dbl_col){n_inputs=1, coeff=[0.00093982], add_latency=1, mult_latency=2, coeff_bit_width=25, coeff_bin_pt=24, first_stage_hdl=on, adder_imp=DSP48}
      mask prompts: n_inputs "Inputs"; coeff "Coefficients"; add_latency "Add latency"; mult_latency "Mult Latency"; coeff_bit_width "Coefficient bit width"; coeff_bin_pt "Coefficient binary point"; first_stage_hdl "Implement first stage of adder trees on output as behavioural HDL"; adder_imp "Adder implementation"
      mask init: same as lo_values_test_v11/dec_fir/fir_dbl_col1
      mask Help: eval('xlWeb(''http://casper.berkeley.edu/wiki/Fir_dbl_col'')')
      mask TypeOptions adder_imp: Behavioral | Fabric | DSP48
  imag_sum : Subsystem  AncestorBlock=casper_library_misc/adder_tree  mask(adder_tree){n_inputs=51, latency=1, adder_imp=DSP48, first_stage_hdl=on}
      mask prompts: n_inputs "Number of Inputs"; latency "Add Latency"; adder_imp "Adder implementation"; first_stage_hdl "Use behavioural HDL for first stage of adders"
      mask help:
      | Sums all inputs using a tree of adds and delays.
      |
      | Number of inputs: The number of inputs to the block to be summed
      | Add latency: The number of clock cycles to perform one addition (affects timing)..
      | Adder implementation: choice of fabric or DSP48E core, or behavioral HDL
      | Use behavioural HDL for first stage of adders: Causes the first stage of adders to be absorbed into DSP blocks if multipliers precede them (Virtex 5). Overrides Adder implementation
      mask init:
      | adder_tree_init(gcb, ...
      |     'n_inputs', n_inputs, ...
      |     'latency', latency, ...
      |     'adder_imp', adder_imp, ...
      |     'first_stage_hdl', first_stage_hdl);
      settings: AttributesFormatString=latency 6
      mask Help: eval('xlWeb(''http://casper.berkeley.edu/wiki/Adder_tree'')')
      mask TypeOptions adder_imp: Behavioral | Fabric | DSP48
  real_sum : Subsystem  AncestorBlock=casper_library_misc/adder_tree  mask(adder_tree){n_inputs=51, latency=1, adder_imp=DSP48, first_stage_hdl=on}
      mask prompts: n_inputs "Number of Inputs"; latency "Add Latency"; adder_imp "Adder implementation"; first_stage_hdl "Use behavioural HDL for first stage of adders"
      mask help:
      | Sums all inputs using a tree of adds and delays.
      |
      | Number of inputs: The number of inputs to the block to be summed
      | Add latency: The number of clock cycles to perform one addition (affects timing)..
      | Adder implementation: choice of fabric or DSP48E core, or behavioral HDL
      | Use behavioural HDL for first stage of adders: Causes the first stage of adders to be absorbed into DSP blocks if multipliers precede them (Virtex 5). Overrides Adder implementation
      mask init:
      | adder_tree_init(gcb, ...
      |     'n_inputs', n_inputs, ...
      |     'latency', latency, ...
      |     'adder_imp', adder_imp, ...
      |     'first_stage_hdl', first_stage_hdl);
      settings: AttributesFormatString=latency 6
      mask Help: eval('xlWeb(''http://casper.berkeley.edu/wiki/Adder_tree'')')
      mask TypeOptions adder_imp: Behavioral | Fabric | DSP48
  ri_to_c : casper_library_misc/ri_to_c
  shift1 : xbsIndex_r4/Shift  shift_dir=Left  shift_bits=1  en=off  latency=0  precision=Full  arith_type="Signed  (2's comp)"  n_bits=16  bin_pt=14  quantization=Truncate  overflow=Wrap  dbl_ovrd=off  block_type=shift
  shift2 : xbsIndex_r4/Shift  shift_dir=Left  shift_bits=1  en=off  latency=0  precision=Full  arith_type="Signed  (2's comp)"  n_bits=16  bin_pt=14  quantization=Truncate  overflow=Wrap  dbl_ovrd=off  block_type=shift
  sync_out : Outport
  dout : Outport  Port=2
  wires:
  real1/1 -> fir_dbl_col1/1(real1)
  imag1/1 -> fir_dbl_col1/2(imag1)
  fir_dbl_col1/5(real_sum) -> real_sum/2(din1)
  fir_dbl_col1/6(imag_sum) -> imag_sum/2(din1)
  fir_dbl_col1/1(real_out1) -> fir_dbl_col2/1(real1)
  fir_dbl_col1/2(imag_out1) -> fir_dbl_col2/2(imag1)
  fir_dbl_col2/5(real_sum) -> real_sum/3(din2)
  fir_dbl_col2/6(imag_sum) -> imag_sum/3(din2)
  fir_dbl_col2/1(real_out1) -> fir_dbl_col3/1(real1)
  fir_dbl_col2/2(imag_out1) -> fir_dbl_col3/2(imag1)
  fir_dbl_col3/5(real_sum) -> real_sum/4(din3)
  fir_dbl_col3/6(imag_sum) -> imag_sum/4(din3)
  fir_dbl_col3/1(real_out1) -> fir_dbl_col4/1(real1)
  fir_dbl_col3/2(imag_out1) -> fir_dbl_col4/2(imag1)
  fir_dbl_col4/5(real_sum) -> real_sum/5(din4)
  fir_dbl_col4/6(imag_sum) -> imag_sum/5(din4)
  fir_dbl_col4/1(real_out1) -> fir_dbl_col5/1(real1)
  fir_dbl_col4/2(imag_out1) -> fir_dbl_col5/2(imag1)
  fir_dbl_col5/5(real_sum) -> real_sum/6(din5)
  fir_dbl_col5/6(imag_sum) -> imag_sum/6(din5)
  fir_dbl_col5/1(real_out1) -> fir_dbl_col6/1(real1)
  fir_dbl_col5/2(imag_out1) -> fir_dbl_col6/2(imag1)
  fir_dbl_col6/5(real_sum) -> real_sum/7(din6)
  fir_dbl_col6/6(imag_sum) -> imag_sum/7(din6)
  fir_dbl_col6/1(real_out1) -> fir_dbl_col7/1(real1)
  fir_dbl_col6/2(imag_out1) -> fir_dbl_col7/2(imag1)
  fir_dbl_col7/5(real_sum) -> real_sum/8(din7)
  fir_dbl_col7/6(imag_sum) -> imag_sum/8(din7)
  fir_dbl_col7/1(real_out1) -> fir_dbl_col8/1(real1)
  fir_dbl_col7/2(imag_out1) -> fir_dbl_col8/2(imag1)
  fir_dbl_col8/5(real_sum) -> real_sum/9(din8)
  fir_dbl_col8/6(imag_sum) -> imag_sum/9(din8)
  fir_dbl_col8/1(real_out1) -> fir_dbl_col9/1(real1)
  fir_dbl_col8/2(imag_out1) -> fir_dbl_col9/2(imag1)
  fir_dbl_col9/5(real_sum) -> real_sum/10(din9)
  fir_dbl_col9/6(imag_sum) -> imag_sum/10(din9)
  fir_dbl_col9/1(real_out1) -> fir_dbl_col10/1(real1)
  fir_dbl_col9/2(imag_out1) -> fir_dbl_col10/2(imag1)
  fir_dbl_col10/5(real_sum) -> real_sum/11(din10)
  fir_dbl_col10/6(imag_sum) -> imag_sum/11(din10)
  fir_dbl_col10/1(real_out1) -> fir_dbl_col11/1(real1)
  fir_dbl_col10/2(imag_out1) -> fir_dbl_col11/2(imag1)
  fir_dbl_col11/5(real_sum) -> real_sum/12(din11)
  fir_dbl_col11/6(imag_sum) -> imag_sum/12(din11)
  fir_dbl_col11/1(real_out1) -> fir_dbl_col12/1(real1)
  fir_dbl_col11/2(imag_out1) -> fir_dbl_col12/2(imag1)
  fir_dbl_col12/5(real_sum) -> real_sum/13(din12)
  fir_dbl_col12/6(imag_sum) -> imag_sum/13(din12)
  fir_dbl_col12/1(real_out1) -> fir_dbl_col13/1(real1)
  fir_dbl_col12/2(imag_out1) -> fir_dbl_col13/2(imag1)
  fir_dbl_col13/5(real_sum) -> real_sum/14(din13)
  fir_dbl_col13/6(imag_sum) -> imag_sum/14(din13)
  fir_dbl_col13/1(real_out1) -> fir_dbl_col14/1(real1)
  fir_dbl_col13/2(imag_out1) -> fir_dbl_col14/2(imag1)
  fir_dbl_col14/5(real_sum) -> real_sum/15(din14)
  fir_dbl_col14/6(imag_sum) -> imag_sum/15(din14)
  fir_dbl_col14/1(real_out1) -> fir_dbl_col15/1(real1)
  fir_dbl_col14/2(imag_out1) -> fir_dbl_col15/2(imag1)
  fir_dbl_col15/5(real_sum) -> real_sum/16(din15)
  fir_dbl_col15/6(imag_sum) -> imag_sum/16(din15)
  fir_dbl_col15/1(real_out1) -> fir_dbl_col16/1(real1)
  fir_dbl_col15/2(imag_out1) -> fir_dbl_col16/2(imag1)
  fir_dbl_col16/5(real_sum) -> real_sum/17(din16)
  fir_dbl_col16/6(imag_sum) -> imag_sum/17(din16)
  fir_dbl_col16/1(real_out1) -> fir_dbl_col17/1(real1)
  fir_dbl_col16/2(imag_out1) -> fir_dbl_col17/2(imag1)
  fir_dbl_col17/5(real_sum) -> real_sum/18(din17)
  fir_dbl_col17/6(imag_sum) -> imag_sum/18(din17)
  fir_dbl_col17/1(real_out1) -> fir_dbl_col18/1(real1)
  fir_dbl_col17/2(imag_out1) -> fir_dbl_col18/2(imag1)
  fir_dbl_col18/5(real_sum) -> real_sum/19(din18)
  fir_dbl_col18/6(imag_sum) -> imag_sum/19(din18)
  fir_dbl_col18/1(real_out1) -> fir_dbl_col19/1(real1)
  fir_dbl_col18/2(imag_out1) -> fir_dbl_col19/2(imag1)
  fir_dbl_col19/5(real_sum) -> real_sum/20(din19)
  fir_dbl_col19/6(imag_sum) -> imag_sum/20(din19)
  fir_dbl_col19/1(real_out1) -> fir_dbl_col20/1(real1)
  fir_dbl_col19/2(imag_out1) -> fir_dbl_col20/2(imag1)
  fir_dbl_col20/5(real_sum) -> real_sum/21(din20)
  fir_dbl_col20/6(imag_sum) -> imag_sum/21(din20)
  fir_dbl_col20/1(real_out1) -> fir_dbl_col21/1(real1)
  fir_dbl_col20/2(imag_out1) -> fir_dbl_col21/2(imag1)
  fir_dbl_col21/5(real_sum) -> real_sum/22(din21)
  fir_dbl_col21/6(imag_sum) -> imag_sum/22(din21)
  fir_dbl_col21/1(real_out1) -> fir_dbl_col22/1(real1)
  fir_dbl_col21/2(imag_out1) -> fir_dbl_col22/2(imag1)
  fir_dbl_col22/5(real_sum) -> real_sum/23(din22)
  fir_dbl_col22/6(imag_sum) -> imag_sum/23(din22)
  fir_dbl_col22/1(real_out1) -> fir_dbl_col23/1(real1)
  fir_dbl_col22/2(imag_out1) -> fir_dbl_col23/2(imag1)
  fir_dbl_col23/5(real_sum) -> real_sum/24(din23)
  fir_dbl_col23/6(imag_sum) -> imag_sum/24(din23)
  fir_dbl_col23/1(real_out1) -> fir_dbl_col24/1(real1)
  fir_dbl_col23/2(imag_out1) -> fir_dbl_col24/2(imag1)
  fir_dbl_col24/5(real_sum) -> real_sum/25(din24)
  fir_dbl_col24/6(imag_sum) -> imag_sum/25(din24)
  fir_dbl_col24/1(real_out1) -> fir_dbl_col25/1(real1)
  fir_dbl_col24/2(imag_out1) -> fir_dbl_col25/2(imag1)
  fir_dbl_col25/5(real_sum) -> real_sum/26(din25)
  fir_dbl_col25/6(imag_sum) -> imag_sum/26(din25)
  fir_dbl_col25/1(real_out1) -> fir_dbl_col26/1(real1)
  fir_dbl_col25/2(imag_out1) -> fir_dbl_col26/2(imag1)
  fir_dbl_col26/5(real_sum) -> real_sum/27(din26)
  fir_dbl_col26/6(imag_sum) -> imag_sum/27(din26)
  fir_dbl_col26/1(real_out1) -> fir_dbl_col27/1(real1)
  fir_dbl_col26/2(imag_out1) -> fir_dbl_col27/2(imag1)
  fir_dbl_col27/5(real_sum) -> real_sum/28(din27)
  fir_dbl_col27/6(imag_sum) -> imag_sum/28(din27)
  fir_dbl_col27/1(real_out1) -> fir_dbl_col28/1(real1)
  fir_dbl_col27/2(imag_out1) -> fir_dbl_col28/2(imag1)
  fir_dbl_col28/5(real_sum) -> real_sum/29(din28)
  fir_dbl_col28/6(imag_sum) -> imag_sum/29(din28)
  fir_dbl_col28/1(real_out1) -> fir_dbl_col29/1(real1)
  fir_dbl_col28/2(imag_out1) -> fir_dbl_col29/2(imag1)
  fir_dbl_col29/5(real_sum) -> real_sum/30(din29)
  fir_dbl_col29/6(imag_sum) -> imag_sum/30(din29)
  fir_dbl_col29/1(real_out1) -> fir_dbl_col30/1(real1)
  fir_dbl_col29/2(imag_out1) -> fir_dbl_col30/2(imag1)
  fir_dbl_col30/5(real_sum) -> real_sum/31(din30)
  fir_dbl_col30/6(imag_sum) -> imag_sum/31(din30)
  fir_dbl_col30/1(real_out1) -> fir_dbl_col31/1(real1)
  fir_dbl_col30/2(imag_out1) -> fir_dbl_col31/2(imag1)
  fir_dbl_col31/5(real_sum) -> real_sum/32(din31)
  fir_dbl_col31/6(imag_sum) -> imag_sum/32(din31)
  fir_dbl_col31/1(real_out1) -> fir_dbl_col32/1(real1)
  fir_dbl_col31/2(imag_out1) -> fir_dbl_col32/2(imag1)
  fir_dbl_col32/5(real_sum) -> real_sum/33(din32)
  fir_dbl_col32/6(imag_sum) -> imag_sum/33(din32)
  fir_dbl_col32/1(real_out1) -> fir_dbl_col33/1(real1)
  fir_dbl_col32/2(imag_out1) -> fir_dbl_col33/2(imag1)
  fir_dbl_col33/5(real_sum) -> real_sum/34(din33)
  fir_dbl_col33/6(imag_sum) -> imag_sum/34(din33)
  fir_dbl_col33/1(real_out1) -> fir_dbl_col34/1(real1)
  fir_dbl_col33/2(imag_out1) -> fir_dbl_col34/2(imag1)
  fir_dbl_col34/5(real_sum) -> real_sum/35(din34)
  fir_dbl_col34/6(imag_sum) -> imag_sum/35(din34)
  fir_dbl_col34/1(real_out1) -> fir_dbl_col35/1(real1)
  fir_dbl_col34/2(imag_out1) -> fir_dbl_col35/2(imag1)
  fir_dbl_col35/5(real_sum) -> real_sum/36(din35)
  fir_dbl_col35/6(imag_sum) -> imag_sum/36(din35)
  fir_dbl_col35/1(real_out1) -> fir_dbl_col36/1(real1)
  fir_dbl_col35/2(imag_out1) -> fir_dbl_col36/2(imag1)
  fir_dbl_col36/5(real_sum) -> real_sum/37(din36)
  fir_dbl_col36/6(imag_sum) -> imag_sum/37(din36)
  fir_dbl_col36/1(real_out1) -> fir_dbl_col37/1(real1)
  fir_dbl_col36/2(imag_out1) -> fir_dbl_col37/2(imag1)
  fir_dbl_col37/5(real_sum) -> real_sum/38(din37)
  fir_dbl_col37/6(imag_sum) -> imag_sum/38(din37)
  fir_dbl_col37/1(real_out1) -> fir_dbl_col38/1(real1)
  fir_dbl_col37/2(imag_out1) -> fir_dbl_col38/2(imag1)
  fir_dbl_col38/5(real_sum) -> real_sum/39(din38)
  fir_dbl_col38/6(imag_sum) -> imag_sum/39(din38)
  fir_dbl_col38/1(real_out1) -> fir_dbl_col39/1(real1)
  fir_dbl_col38/2(imag_out1) -> fir_dbl_col39/2(imag1)
  fir_dbl_col39/5(real_sum) -> real_sum/40(din39)
  fir_dbl_col39/6(imag_sum) -> imag_sum/40(din39)
  fir_dbl_col39/1(real_out1) -> fir_dbl_col40/1(real1)
  fir_dbl_col39/2(imag_out1) -> fir_dbl_col40/2(imag1)
  fir_dbl_col40/5(real_sum) -> real_sum/41(din40)
  fir_dbl_col40/6(imag_sum) -> imag_sum/41(din40)
  fir_dbl_col40/1(real_out1) -> fir_dbl_col41/1(real1)
  fir_dbl_col40/2(imag_out1) -> fir_dbl_col41/2(imag1)
  fir_dbl_col41/5(real_sum) -> real_sum/42(din41)
  fir_dbl_col41/6(imag_sum) -> imag_sum/42(din41)
  fir_dbl_col41/1(real_out1) -> fir_dbl_col42/1(real1)
  fir_dbl_col41/2(imag_out1) -> fir_dbl_col42/2(imag1)
  fir_dbl_col42/5(real_sum) -> real_sum/43(din42)
  fir_dbl_col42/6(imag_sum) -> imag_sum/43(din42)
  fir_dbl_col42/1(real_out1) -> fir_dbl_col43/1(real1)
  fir_dbl_col42/2(imag_out1) -> fir_dbl_col43/2(imag1)
  fir_dbl_col43/5(real_sum) -> real_sum/44(din43)
  fir_dbl_col43/6(imag_sum) -> imag_sum/44(din43)
  fir_dbl_col43/1(real_out1) -> fir_dbl_col44/1(real1)
  fir_dbl_col43/2(imag_out1) -> fir_dbl_col44/2(imag1)
  fir_dbl_col44/5(real_sum) -> real_sum/45(din44)
  fir_dbl_col44/6(imag_sum) -> imag_sum/45(din44)
  fir_dbl_col44/1(real_out1) -> fir_dbl_col45/1(real1)
  fir_dbl_col44/2(imag_out1) -> fir_dbl_col45/2(imag1)
  fir_dbl_col45/5(real_sum) -> real_sum/46(din45)
  fir_dbl_col45/6(imag_sum) -> imag_sum/46(din45)
  fir_dbl_col45/1(real_out1) -> fir_dbl_col46/1(real1)
  fir_dbl_col45/2(imag_out1) -> fir_dbl_col46/2(imag1)
  fir_dbl_col46/5(real_sum) -> real_sum/47(din46)
  fir_dbl_col46/6(imag_sum) -> imag_sum/47(din46)
  fir_dbl_col46/1(real_out1) -> fir_dbl_col47/1(real1)
  fir_dbl_col46/2(imag_out1) -> fir_dbl_col47/2(imag1)
  fir_dbl_col47/5(real_sum) -> real_sum/48(din47)
  fir_dbl_col47/6(imag_sum) -> imag_sum/48(din47)
  fir_dbl_col47/1(real_out1) -> fir_dbl_col48/1(real1)
  fir_dbl_col47/2(imag_out1) -> fir_dbl_col48/2(imag1)
  fir_dbl_col48/5(real_sum) -> real_sum/49(din48)
  fir_dbl_col48/6(imag_sum) -> imag_sum/49(din48)
  fir_dbl_col48/1(real_out1) -> fir_dbl_col49/1(real1)
  fir_dbl_col48/2(imag_out1) -> fir_dbl_col49/2(imag1)
  fir_dbl_col49/5(real_sum) -> real_sum/50(din49)
  fir_dbl_col49/6(imag_sum) -> imag_sum/50(din49)
  fir_dbl_col49/1(real_out1) -> fir_dbl_col50/1(real1)
  fir_dbl_col49/2(imag_out1) -> fir_dbl_col50/2(imag1)
  fir_dbl_col50/5(real_sum) -> real_sum/51(din50)
  fir_dbl_col50/6(imag_sum) -> imag_sum/51(din50)
  fir_dbl_col50/1(real_out1) -> fir_dbl_col51/1(real1)
  fir_dbl_col50/2(imag_out1) -> fir_dbl_col51/2(imag1)
  fir_dbl_col51/5(real_sum) -> real_sum/52(din51)
  fir_dbl_col51/6(imag_sum) -> imag_sum/52(din51)
  real_sum/2(dout) -> shift1/1
  imag_sum/2(dout) -> shift2/1
  shift1/1 -> convert1/1
  shift2/1 -> convert2/1
  convert1/1 -> ri_to_c/1
  convert2/1 -> ri_to_c/2
  ri_to_c/1 -> dout/1
  sync_in/1 -> delay/1
  delay/1 -> real_sum/1(sync), imag_sum/1(sync)
  real_sum/1(sync_out) -> sync_out/1
  fir_dbl_col2/3(real_back_out1) -> fir_dbl_col1/3(real_back1)
  fir_dbl_col2/4(imag_back_out1) -> fir_dbl_col1/4(imag_back1)
  fir_dbl_col3/3(real_back_out1) -> fir_dbl_col2/3(real_back1)
  fir_dbl_col3/4(imag_back_out1) -> fir_dbl_col2/4(imag_back1)
  fir_dbl_col4/3(real_back_out1) -> fir_dbl_col3/3(real_back1)
  fir_dbl_col4/4(imag_back_out1) -> fir_dbl_col3/4(imag_back1)
  fir_dbl_col5/3(real_back_out1) -> fir_dbl_col4/3(real_back1)
  fir_dbl_col5/4(imag_back_out1) -> fir_dbl_col4/4(imag_back1)
  fir_dbl_col6/3(real_back_out1) -> fir_dbl_col5/3(real_back1)
  fir_dbl_col6/4(imag_back_out1) -> fir_dbl_col5/4(imag_back1)
  fir_dbl_col7/3(real_back_out1) -> fir_dbl_col6/3(real_back1)
  fir_dbl_col7/4(imag_back_out1) -> fir_dbl_col6/4(imag_back1)
  fir_dbl_col8/3(real_back_out1) -> fir_dbl_col7/3(real_back1)
  fir_dbl_col8/4(imag_back_out1) -> fir_dbl_col7/4(imag_back1)
  fir_dbl_col9/3(real_back_out1) -> fir_dbl_col8/3(real_back1)
  fir_dbl_col9/4(imag_back_out1) -> fir_dbl_col8/4(imag_back1)
  fir_dbl_col10/3(real_back_out1) -> fir_dbl_col9/3(real_back1)
  fir_dbl_col10/4(imag_back_out1) -> fir_dbl_col9/4(imag_back1)
  fir_dbl_col11/3(real_back_out1) -> fir_dbl_col10/3(real_back1)
  fir_dbl_col11/4(imag_back_out1) -> fir_dbl_col10/4(imag_back1)
  fir_dbl_col12/3(real_back_out1) -> fir_dbl_col11/3(real_back1)
  fir_dbl_col12/4(imag_back_out1) -> fir_dbl_col11/4(imag_back1)
  fir_dbl_col13/3(real_back_out1) -> fir_dbl_col12/3(real_back1)
  fir_dbl_col13/4(imag_back_out1) -> fir_dbl_col12/4(imag_back1)
  fir_dbl_col14/3(real_back_out1) -> fir_dbl_col13/3(real_back1)
  fir_dbl_col14/4(imag_back_out1) -> fir_dbl_col13/4(imag_back1)
  fir_dbl_col15/3(real_back_out1) -> fir_dbl_col14/3(real_back1)
  fir_dbl_col15/4(imag_back_out1) -> fir_dbl_col14/4(imag_back1)
  fir_dbl_col16/3(real_back_out1) -> fir_dbl_col15/3(real_back1)
  fir_dbl_col16/4(imag_back_out1) -> fir_dbl_col15/4(imag_back1)
  fir_dbl_col17/3(real_back_out1) -> fir_dbl_col16/3(real_back1)
  fir_dbl_col17/4(imag_back_out1) -> fir_dbl_col16/4(imag_back1)
  fir_dbl_col18/3(real_back_out1) -> fir_dbl_col17/3(real_back1)
  fir_dbl_col18/4(imag_back_out1) -> fir_dbl_col17/4(imag_back1)
  fir_dbl_col19/3(real_back_out1) -> fir_dbl_col18/3(real_back1)
  fir_dbl_col19/4(imag_back_out1) -> fir_dbl_col18/4(imag_back1)
  fir_dbl_col20/3(real_back_out1) -> fir_dbl_col19/3(real_back1)
  fir_dbl_col20/4(imag_back_out1) -> fir_dbl_col19/4(imag_back1)
  fir_dbl_col21/3(real_back_out1) -> fir_dbl_col20/3(real_back1)
  fir_dbl_col21/4(imag_back_out1) -> fir_dbl_col20/4(imag_back1)
  fir_dbl_col22/3(real_back_out1) -> fir_dbl_col21/3(real_back1)
  fir_dbl_col22/4(imag_back_out1) -> fir_dbl_col21/4(imag_back1)
  fir_dbl_col23/3(real_back_out1) -> fir_dbl_col22/3(real_back1)
  fir_dbl_col23/4(imag_back_out1) -> fir_dbl_col22/4(imag_back1)
  fir_dbl_col24/3(real_back_out1) -> fir_dbl_col23/3(real_back1)
  fir_dbl_col24/4(imag_back_out1) -> fir_dbl_col23/4(imag_back1)
  fir_dbl_col25/3(real_back_out1) -> fir_dbl_col24/3(real_back1)
  fir_dbl_col25/4(imag_back_out1) -> fir_dbl_col24/4(imag_back1)
  fir_dbl_col26/3(real_back_out1) -> fir_dbl_col25/3(real_back1)
  fir_dbl_col26/4(imag_back_out1) -> fir_dbl_col25/4(imag_back1)
  fir_dbl_col27/3(real_back_out1) -> fir_dbl_col26/3(real_back1)
  fir_dbl_col27/4(imag_back_out1) -> fir_dbl_col26/4(imag_back1)
  fir_dbl_col28/3(real_back_out1) -> fir_dbl_col27/3(real_back1)
  fir_dbl_col28/4(imag_back_out1) -> fir_dbl_col27/4(imag_back1)
  fir_dbl_col29/3(real_back_out1) -> fir_dbl_col28/3(real_back1)
  fir_dbl_col29/4(imag_back_out1) -> fir_dbl_col28/4(imag_back1)
  fir_dbl_col30/3(real_back_out1) -> fir_dbl_col29/3(real_back1)
  fir_dbl_col30/4(imag_back_out1) -> fir_dbl_col29/4(imag_back1)
  fir_dbl_col31/3(real_back_out1) -> fir_dbl_col30/3(real_back1)
  fir_dbl_col31/4(imag_back_out1) -> fir_dbl_col30/4(imag_back1)
  fir_dbl_col32/3(real_back_out1) -> fir_dbl_col31/3(real_back1)
  fir_dbl_col32/4(imag_back_out1) -> fir_dbl_col31/4(imag_back1)
  fir_dbl_col33/3(real_back_out1) -> fir_dbl_col32/3(real_back1)
  fir_dbl_col33/4(imag_back_out1) -> fir_dbl_col32/4(imag_back1)
  fir_dbl_col34/3(real_back_out1) -> fir_dbl_col33/3(real_back1)
  fir_dbl_col34/4(imag_back_out1) -> fir_dbl_col33/4(imag_back1)
  fir_dbl_col35/3(real_back_out1) -> fir_dbl_col34/3(real_back1)
  fir_dbl_col35/4(imag_back_out1) -> fir_dbl_col34/4(imag_back1)
  fir_dbl_col36/3(real_back_out1) -> fir_dbl_col35/3(real_back1)
  fir_dbl_col36/4(imag_back_out1) -> fir_dbl_col35/4(imag_back1)
  fir_dbl_col37/3(real_back_out1) -> fir_dbl_col36/3(real_back1)
  fir_dbl_col37/4(imag_back_out1) -> fir_dbl_col36/4(imag_back1)
  fir_dbl_col38/3(real_back_out1) -> fir_dbl_col37/3(real_back1)
  fir_dbl_col38/4(imag_back_out1) -> fir_dbl_col37/4(imag_back1)
  fir_dbl_col39/3(real_back_out1) -> fir_dbl_col38/3(real_back1)
  fir_dbl_col39/4(imag_back_out1) -> fir_dbl_col38/4(imag_back1)
  fir_dbl_col40/3(real_back_out1) -> fir_dbl_col39/3(real_back1)
  fir_dbl_col40/4(imag_back_out1) -> fir_dbl_col39/4(imag_back1)
  fir_dbl_col41/3(real_back_out1) -> fir_dbl_col40/3(real_back1)
  fir_dbl_col41/4(imag_back_out1) -> fir_dbl_col40/4(imag_back1)
  fir_dbl_col42/3(real_back_out1) -> fir_dbl_col41/3(real_back1)
  fir_dbl_col42/4(imag_back_out1) -> fir_dbl_col41/4(imag_back1)
  fir_dbl_col43/3(real_back_out1) -> fir_dbl_col42/3(real_back1)
  fir_dbl_col43/4(imag_back_out1) -> fir_dbl_col42/4(imag_back1)
  fir_dbl_col44/3(real_back_out1) -> fir_dbl_col43/3(real_back1)
  fir_dbl_col44/4(imag_back_out1) -> fir_dbl_col43/4(imag_back1)
  fir_dbl_col45/3(real_back_out1) -> fir_dbl_col44/3(real_back1)
  fir_dbl_col45/4(imag_back_out1) -> fir_dbl_col44/4(imag_back1)
  fir_dbl_col46/3(real_back_out1) -> fir_dbl_col45/3(real_back1)
  fir_dbl_col46/4(imag_back_out1) -> fir_dbl_col45/4(imag_back1)
  fir_dbl_col47/3(real_back_out1) -> fir_dbl_col46/3(real_back1)
  fir_dbl_col47/4(imag_back_out1) -> fir_dbl_col46/4(imag_back1)
  fir_dbl_col48/3(real_back_out1) -> fir_dbl_col47/3(real_back1)
  fir_dbl_col48/4(imag_back_out1) -> fir_dbl_col47/4(imag_back1)
  fir_dbl_col49/3(real_back_out1) -> fir_dbl_col48/3(real_back1)
  fir_dbl_col49/4(imag_back_out1) -> fir_dbl_col48/4(imag_back1)
  fir_dbl_col50/3(real_back_out1) -> fir_dbl_col49/3(real_back1)
  fir_dbl_col50/4(imag_back_out1) -> fir_dbl_col49/4(imag_back1)
  fir_dbl_col51/3(real_back_out1) -> fir_dbl_col50/3(real_back1)
  fir_dbl_col51/4(imag_back_out1) -> fir_dbl_col50/4(imag_back1)
  fir_dbl_col51/1(real_out1) -> fir_dbl_col51/3(real_back1)
  fir_dbl_col51/2(imag_out1) -> fir_dbl_col51/4(imag_back1)
